simulink subsystem "Day3_Scenario_1"  (R2024a)
settings: Solver=VariableStepAuto  StartTime=0.0  StopTime=10.0  RelTol=1e-3
undefined symbols (not defined in the file): left_first_line_point_x, right_first_line_point_x
libraries: CarMaker4SL x6, slpidlib x1
settings Model: Creator=junhyung.cha  LastModifiedBy=pc

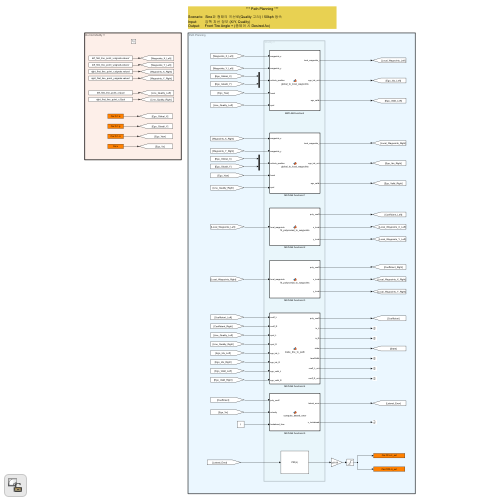
[thumbnail: Simulink's stored preview of the top-level diagram]
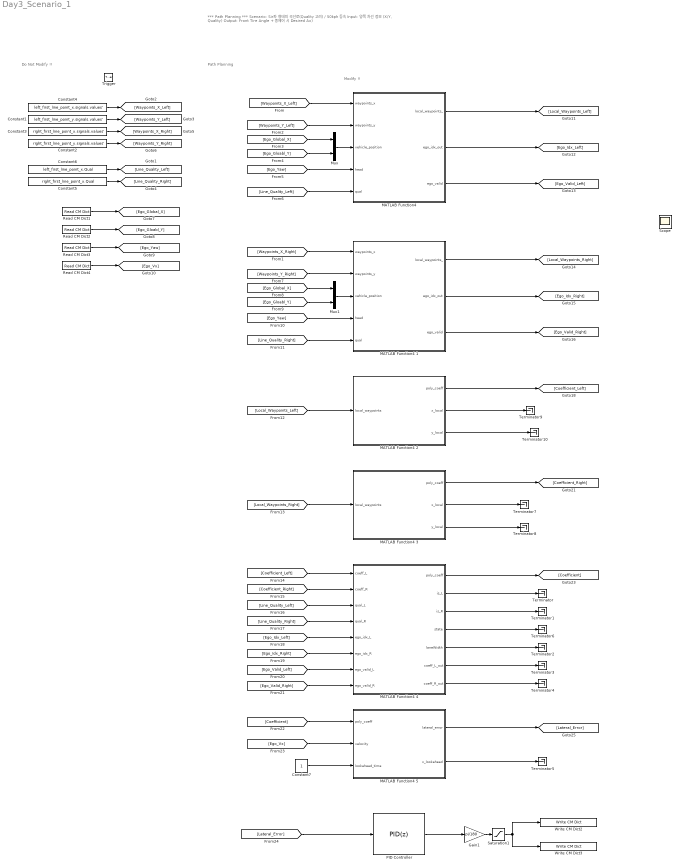
== system Day3_Scenario_1 ==
  note: Path Planning
  note: Do Not Modify !!
  note: Modify !!
  note: *** Path Planning ***
      |
      | Scenario: Sine파 형태의 곡선로(Quality 고려) / 50kph 등속
      | Input: 양쪽 차선 정보 (X/Y, Quality)
      | Output: Front Tire Angle + (종제어 시 Desired Ax)
  Trigger : TriggerPort  TriggerType=function-call  VariantControl=(inherit)
  Constant1 : Constant  Value=left_first_line_point_y.signals.values'
  Constant2 : Constant  Value=right_first_line_point_y.signals.values'
  Constant3 : Constant  Value=right_first_line_point_x.signals.values'
  Constant4 : Constant  Value=left_first_line_point_x.signals.values'
  Constant5 : Constant  Value=right_first_line_point_x.Qual
  Constant6 : Constant  Value=left_first_line_point_x.Qual
  Constant7 : Constant
  Gain1 : Gain  Gain=pi/180
  "MATLAB Function4 " : MATLAB Function  TreatAsAtomicUnit=on
  MATLAB Function4 1 : MATLAB Function  TreatAsAtomicUnit=on
  MATLAB Function4 2 : MATLAB Function  TreatAsAtomicUnit=on
  MATLAB Function4 3 : MATLAB Function  TreatAsAtomicUnit=on
  MATLAB Function4 4 : MATLAB Function  TreatAsAtomicUnit=on
  MATLAB Function4 5 : MATLAB Function  TreatAsAtomicUnit=on
  Mux : Mux  Inputs=2
  Mux1 : Mux  Inputs=2
  PID Controller : slpidlib/PID Controller  Controller=PID  Form=Parallel  TimeDomain=Discrete-time  UseExternalTs=off  SampleTime=-1  IntegratorMethod=Forward Euler  FilterMethod=Forward Euler  ControllerParametersSource=internal  P=0.201  I=0  UseKiTs=off  D=0.0001  UseExternalDerivativeSource=off  N=100  UseFilter=off  TunerSelectOption=Transfer Function Based (PID Tuner App)  InitialConditionSource=internal  InitialConditionForIntegrator=0  InitialConditionForFilter=0  DifferentiatorICPrevScaledInput=0  ExternalReset=none  TrackingMode=off  Kt=1  LimitOutput=off  SatLimitsSource=internal  UpperSaturationLimit=inf  LowerSaturationLimit=-inf  LinearizeAsGain=on  AntiWindupMode=none  Kb=1  LimitIntegrator=off  UpperIntegratorSaturationLimit=inf  LowerIntegratorSaturationLimit=-inf  POutMin=[]  POutMax=[]  IOutMin=[]  IOutMax=[]  DOutMin=[]  DOutMax=[]  NOutMin=[]  NOutMax=[]  SumOutMin=[]  SumOutMax=[]  SaturationOutMin=[]  SaturationOutMax=[]  PParamMin=[]  PParamMax=[]  IParamMin=[]  IParamMax=[]  DParamMin=[]  DParamMax=[]  NParamMin=[]  NParamMax=[]  KbParamMin=[]  KbParamMax=[]  KtParamMin=[]  KtParamMax=[]  KbOutMin=[]  KbOutMax=[]  KtOutMin=[]  KtOutMax=[]  IntegratorOutMin=[]  IntegratorOutMax=[]  FilterOutMin=[]  FilterOutMax=[]  SumI1OutMin=[]  SumI1OutMax=[]  SumI2OutMin=[]  SumI2OutMax=[]  SumI3OutMin=[]  SumI3OutMax=[]  SumI4OutMin=[]  SumI4OutMax=[]  SumDOutMin=[]  SumDOutMax=[]  DifferentiatorOutMin=[]  DifferentiatorOutMax=[]  FilterDiffOutCoefMin=[]  FilterDiffOutCoefMax=[]  ReciprocalOutMin=[]  ReciprocalOutMax=[]  SumDenOutMin=[]  SumDenOutMax=[]  SumNumOutMin=[]  SumNumOutMax=[]  DivideOutMin=[]  DivideOutMax=[]  UdiffTsProdOutMin=[]  UdiffTsProdOutMax=[]  NTsProdOutMin=[]  NTsProdOutMax=[]  UintegralTsProdOutMin=[]  UintegralTsProdOutMax=[]  UngainTsProdOutMin=[]  UngainTsProdOutMax=[]  ClampingZeroOutDataTypeStr=Inherit: Inherit via back propagation  ClampingZeroOutMin=[]  ClampingZeroOutMax=[]  FilterDenConstantOutDataTypeStr=Inherit: Inherit via back propagation  FilterDenConstantOutMin=[]  FilterDenConstantOutMax=[]  PCopyOutDataTypeStr=Inherit: Inherit via back propagation  PCopyOutMin=[]  PCopyOutMax=[]  NCopyOutDataTypeStr=Inherit: Inherit via back propagation  NCopyOutMin=[]  NCopyOutMax=[]  IntegratorContinuousStateAttributes=''  IntegratorStateMustResolveToSignalObject=off  IntegratorRTWStateStorageClass=Auto  FilterContinuousStateAttributes=''  FilterStateMustResolveToSignalObject=off  FilterRTWStateStorageClass=Auto  ParallelPVariant=InternalParameters  IdealPVariant=Disabled  IVariant=InternalParameters  DVariant=InternalParameters  IntegratorVariant=Discrete  SatVariant=Disabled  AWVariant=Passthrough  PCopyVariant=Disabled  TRVariant=Disabled  FdbkBlocksVariant=Forward  IdealPFdbkVariant=Disabled  SatFdbkVariant=Disabled  DerivativeFilterVariant=Differentiator  NVariant=Passthrough  NCopyVariant=Disabled_SignalSpec  FilterICVariant=InternalICsDifferentiator  IntegratorICVariant=InternalICs  ExternalResetVariant=Disabled  TRSumVariant=Passthrough  SumFdbkVariant=Disabled  SumVariant=Sum_PID  TsampFilterVariant=InternalTs  TsampNgainVariant=Passthrough  TsampIntegralVariant=Disabled_SignalSpec  ExternalSaturationOutDataTypeStr=Inherit: Same as second input  DerivativeSourceVariant=ErrorSignal
  Read CM Dict1 : CarMaker4SL/Read CM Dict  xname=Car.Fr1.tx  xsync=off  xstime=Inherited
  Read CM Dict2 : CarMaker4SL/Read CM Dict  xname=Car.Fr1.ty  xsync=off  xstime=Inherited
  Read CM Dict3 : CarMaker4SL/Read CM Dict  xname=Car.Fr1.rz  xsync=off  xstime=Inherited
  Read CM Dict4 : CarMaker4SL/Read CM Dict  xname=Car.v  xsync=off  xstime=Inherited
  Saturation1 : Saturate  UpperLimit=2  LowerLimit=-2
  Scope : Scope
  Terminator{,1..10} (11 alike) : Terminator
  Write CM Dict2 : CarMaker4SL/Write CM Dict  xname=Car.CFL.rz_ext  xsync=off
  Write CM Dict3 : CarMaker4SL/Write CM Dict  xname=Car.CFR.rz_ext  xsync=off
  wires:
  Constant4/1 -> [Waypoints_X_Left]
  Constant1/1 -> [Waypoints_Y_Left]
  Constant2/1 -> [Waypoints_Y_Right]
  Constant3/1 -> [Waypoints_X_Right]
  [Waypoints_X_Left] -> "MATLAB Function4 "/1(waypoints_x)
  [Waypoints_Y_Left] -> "MATLAB Function4 "/2(waypoints_y)
  Mux/1 -> "MATLAB Function4 "/3(vehicle_position)
  [Ego_Global_X] -> Mux/1
  Read CM Dict2/1 -> [Ego_Gloabl_Y]
  Read CM Dict1/1 -> [Ego_Global_X]
  [Ego_Gloabl_Y] -> Mux/2
  Read CM Dict3/1 -> [Ego_Yaw]
  [Ego_Yaw] -> "MATLAB Function4 "/4(head)
  Constant5/1 -> [Line_Quality_Right]
  Constant6/1 -> [Line_Quality_Left]
  [Line_Quality_Left] -> "MATLAB Function4 "/5(qual)
  [Line_Quality_Right] -> MATLAB Function4 1/5(qual)
  [Ego_Yaw] -> MATLAB Function4 1/4(head)
  [Ego_Gloabl_Y] -> Mux1/2
  [Ego_Global_X] -> Mux1/1
  [Waypoints_Y_Right] -> MATLAB Function4 1/2(waypoints_y)
  [Waypoints_X_Right] -> MATLAB Function4 1/1(waypoints_x)
  Mux1/1 -> MATLAB Function4 1/3(vehicle_position)
  "MATLAB Function4 "/3(ego_valid) -> [Ego_Valid_Left]
  "MATLAB Function4 "/2(ego_idx_out) -> [Ego_Idx_Left]
  "MATLAB Function4 "/1(local_waypoints_) -> [Local_Waypoints_Left]
  MATLAB Function4 1/1(local_waypoints_) -> [Local_Waypoints_Right]
  MATLAB Function4 1/2(ego_idx_out) -> [Ego_Idx_Right]
  MATLAB Function4 1/3(ego_valid) -> [Ego_Valid_Right]
  [Local_Waypoints_Left] -> MATLAB Function4 2/1(local_waypoints)
  [Local_Waypoints_Right] -> MATLAB Function4 3/1(local_waypoints)
  MATLAB Function4 2/1(poly_coeff) -> [Coefficient_Left]
  MATLAB Function4 2/2(x_local) -> Terminator9/1
  MATLAB Function4 2/3(y_local) -> Terminator10/1
  MATLAB Function4 3/3(y_local) -> Terminator8/1
  MATLAB Function4 3/2(x_local) -> Terminator7/1
  MATLAB Function4 3/1(poly_coeff) -> [Coefficient_Right]
  MATLAB Function4 4/1(poly_coeff) -> [Coefficient]
  MATLAB Function4 4/4(state) -> Terminator6/1
  MATLAB Function4 4/2(is_L) -> Terminator/1
  MATLAB Function4 4/3(is_R) -> Terminator1/1
  MATLAB Function4 4/6(coeff_L_out) -> Terminator3/1
  MATLAB Function4 4/5(laneWidth) -> Terminator2/1
  MATLAB Function4 4/7(coeff_R_out) -> Terminator4/1
  [Coefficient] -> MATLAB Function4 5/1(poly_coeff)
  Read CM Dict4/1 -> [Ego_Vx]
  [Ego_Vx] -> MATLAB Function4 5/2(velocity)
  Constant7/1 -> MATLAB Function4 5/3(lookahead_time)
  Saturation1/1 -> Write CM Dict3/1, Write CM Dict2/1
  Gain1/1 -> Saturation1/1
  MATLAB Function4 5/1(lateral_error) -> [Lateral_Error]
  MATLAB Function4 5/2(x_lookahead) -> Terminator5/1
  [Lateral_Error] -> PID Controller/1
  PID Controller/1 -> Gain1/1
  [Coefficient_Left] -> MATLAB Function4 4/1(coeff_L)
  [Coefficient_Right] -> MATLAB Function4 4/2(coeff_R)
  [Line_Quality_Left] -> MATLAB Function4 4/3(qual_L)
  [Line_Quality_Right] -> MATLAB Function4 4/4(qual_R)
  [Ego_Idx_Left] -> MATLAB Function4 4/5(ego_idx_L)
  [Ego_Idx_Right] -> MATLAB Function4 4/6(ego_idx_R)
  [Ego_Valid_Left] -> MATLAB Function4 4/7(ego_valid_L)
  [Ego_Valid_Right] -> MATLAB Function4 4/8(ego_valid_R)

== matlab function Day3_Scenario_1/MATLAB Function4  ==
  settings: sampleTime=0.1
  data: waypoints_x input; waypoints_y input; local_waypoints_ output; vehicle_position input; head input; qual input; ego_idx_out output; ego_valid output
function [local_waypoints_, ego_idx_out, ego_valid] = global_to_local_waypoints_left(waypoints_x, waypoints_y, vehicle_position, head, qual)
    % 우측 차선 전역 → 로컬 좌표 변환 및 유효 인덱스 계산

    N = numel(waypoints_x);
    local_waypoints_ = zeros(N, 2);

    % 차량 yaw 방향의 회전 행렬 파라미터
    cos_h = cos(head);
    sin_h = sin(head);

    % 1) 전역 좌표 → 로컬 좌표
    for i = 1:N
        dx = waypoints_x(i) - vehicle_position(1);
        dy = waypoints_y(i) - vehicle_position(2);
        % (x', y') = R(-head) * [dx; dy]
        x_local =  dx * cos_h + dy * sin_h;
        y_local = -dx * sin_h + dy * cos_h;
        local_waypoints_(i, :) = [x_local, y_local];
    end

    % 2) qual == 1 (유효)인 인덱스들만 추출
    valid_indices = find(qual == 1);

    % 파라미터: 최대 인식 거리
    max_distance = 30; % meter

    % 3) 유효 지점 중 전방 x_local 거리 기준 최소값 선택 (30m 이내만)
    if ~isempty(valid_indices)
        x_vals = local_waypoints_(valid_indices, 1);
        d_vals = abs(x_vals);  % 전방 거리 기준
        d_vals(x_vals < 0 | d_vals > max_distance) = Inf;  % 후방 또는 너무 먼 점 제거

        [~, idx_min] = min(d_vals);
        if isinf(d_vals(idx_min))
            ego_idx_out = -1;
            ego_valid   = 0;
        else
            ego_idx_out = valid_indices(idx_min);
            ego_valid   = 1;
        end
    else
        ego_idx_out = -1;
        ego_valid   = 0;
    end
end

== matlab function Day3_Scenario_1/MATLAB Function4 1 ==
  settings: sampleTime=0.1
  data: waypoints_x input; waypoints_y input; local_waypoints_ output; vehicle_position input; head input; qual input; ego_idx_out output; ego_valid output
function [local_waypoints_, ego_idx_out, ego_valid] = global_to_local_waypoints_left(waypoints_x, waypoints_y, vehicle_position, head, qual)
    % 우측 차선 전역 → 로컬 좌표 변환 및 유효 인덱스 계산

    N = numel(waypoints_x);
    local_waypoints_ = zeros(N, 2);

    % 차량 yaw 방향의 회전 행렬 파라미터
    cos_h = cos(head);
    sin_h = sin(head);

    % 1) 전역 좌표 → 로컬 좌표
    for i = 1:N
        dx = waypoints_x(i) - vehicle_position(1);
        dy = waypoints_y(i) - vehicle_position(2);
        % (x', y') = R(-head) * [dx; dy]
        x_local =  dx * cos_h + dy * sin_h;
        y_local = -dx * sin_h + dy * cos_h;
        local_waypoints_(i, :) = [x_local, y_local];
    end

    % 2) qual == 1 (유효)인 인덱스들만 추출
    valid_indices = find(qual == 1);

    % 파라미터: 최대 인식 거리
    max_distance = 30; % meter

    % 3) 유효 지점 중 전방 x_local 거리 기준 최소값 선택 (30m 이내만)
    if ~isempty(valid_indices)
        x_vals = local_waypoints_(valid_indices, 1);
        d_vals = abs(x_vals);  % 전방 거리 기준
        d_vals(x_vals < 0 | d_vals > max_distance) = Inf;  % 후방 또는 너무 먼 점 제거

        [~, idx_min] = min(d_vals);
        if isinf(d_vals(idx_min))
            ego_idx_out = -1;
            ego_valid   = 0;
        else
            ego_idx_out = valid_indices(idx_min);
            ego_valid   = 1;
        end
    else
        ego_idx_out = -1;
        ego_valid   = 0;
    end
end

== matlab function Day3_Scenario_1/MATLAB Function4 2 ==
  settings: sampleTime=0.1
  data: local_waypoints input; poly_coeff output; x_local output; y_local output
function [poly_coeff, x_local, y_local] = fit_polynomial_to_waypoints(local_waypoints)
%#codegen
% Sliding-Window 기반 3차 다항식 피팅 + Fallback 구현
%
% local_waypoints : Nx2 [x y] in vehicle-local frame
% poly_coeff      : 1x4 [a3 a2 a1 a0]
% x_local, y_local: MAX_POINTS×1 윈도우에 저장된 값 (나머지는 0)

    %% 파라미터
    MAX_DIST   = 15.0;    % 전방 최대 거리 [m]
    MAX_POINTS = 11;      % 최대 포인트 개수
    MAX_ORDER  = 3;       % 최대 다항식 차수

    %% persistent Fallback 변수
    persistent prev_poly prev_kappa prev_laneWidth
    if isempty(prev_poly)
        prev_poly      = zeros(1, MAX_ORDER+1);
        prev_kappa     = 0;
        prev_laneWidth = 3.5;
    end

    %% 출력 초기화
    poly_coeff = zeros(1, MAX_ORDER+1);
    x_local    = zeros(MAX_POINTS,1);
    y_local    = zeros(MAX_POINTS,1);

    %% 1) 전방 필터링 + 윈도우 저장
    stored = 0;
    x_all  = local_waypoints(:,1);
    y_all  = local_waypoints(:,2);
    for i = 1:length(x_all)
        if x_all(i) > 0 && x_all(i) < MAX_DIST
            if stored < MAX_POINTS
                stored = stored + 1;
                x_local(stored) = x_all(i);
                y_local(stored) = y_all(i);
            end
        end
    end

    %% 2) 충분한 점 + 다양한 x 값 체크
    unique_x = numel(unique(x_local(1:stored)));
    if stored < 2 || unique_x < 2
        % 웨이포인트 부족 시 Fallback
        poly_coeff = prev_poly;
        return;
    end

    %% 3) 적정 차수 결정 (점 수에 따라 자동 축소)
    deg = min([MAX_ORDER, stored-1, unique_x-1]);

    %% 4) 정규화된 polyfit 호출
    [p, S, mu] = polyfit(x_local(1:stored), y_local(1:stored), deg);

    %% 5) 조건 수 확인 및 차수 재조정(Optional)
    if isfield(S, 'R')
        if cond(S.R) > 1e6 && deg > 1
            deg = deg - 1;
            [p, S, mu] = polyfit(x_local(1:stored), y_local(1:stored), deg);
        end
    end

    %% 6) 결과 확장 및 출력
    poly_coeff = zeros(1, MAX_ORDER+1);
    poly_coeff(end-deg:end) = p;

    %% 7) Fallback 상태 저장
    % 곡률 계산 (간단히 lookahead x=velocity*dt 등은 상위 로직에서)
    % 여기서는 poly_coeff 저장만
    prev_poly      = poly_coeff;
    % prev_kappa, prev_laneWidth 는 상위 모듈에서 업데이트
end

== matlab function Day3_Scenario_1/MATLAB Function4 3 ==
  settings: sampleTime=0.1
  data: local_waypoints input; poly_coeff output; x_local output; y_local output
function [poly_coeff, x_local, y_local] = fit_polynomial_to_waypoints(local_waypoints)
%#codegen
% Sliding-Window 기반 3차 다항식 피팅 + Fallback 구현
%
% local_waypoints : Nx2 [x y] in vehicle-local frame
% poly_coeff      : 1x4 [a3 a2 a1 a0]
% x_local, y_local: MAX_POINTS×1 윈도우에 저장된 값 (나머지는 0)

    %% 파라미터
    MAX_DIST   = 15.0;    % 전방 최대 거리 [m]
    MAX_POINTS = 11;      % 최대 포인트 개수
    MAX_ORDER  = 3;       % 최대 다항식 차수

    %% persistent Fallback 변수
    persistent prev_poly prev_kappa prev_laneWidth
    if isempty(prev_poly)
        prev_poly      = zeros(1, MAX_ORDER+1);
        prev_kappa     = 0;
        prev_laneWidth = 3.5;
    end

    %% 출력 초기화
    poly_coeff = zeros(1, MAX_ORDER+1);
    x_local    = zeros(MAX_POINTS,1);
    y_local    = zeros(MAX_POINTS,1);

    %% 1) 전방 필터링 + 윈도우 저장
    stored = 0;
    x_all  = local_waypoints(:,1);
    y_all  = local_waypoints(:,2);
    for i = 1:length(x_all)
        if x_all(i) > 0 && x_all(i) < MAX_DIST
            if stored < MAX_POINTS
                stored = stored + 1;
                x_local(stored) = x_all(i);
                y_local(stored) = y_all(i);
            end
        end
    end

    %% 2) 충분한 점 + 다양한 x 값 체크
    unique_x = numel(unique(x_local(1:stored)));
    if stored < 2 || unique_x < 2
        % 웨이포인트 부족 시 Fallback
        poly_coeff = prev_poly;
        return;
    end

    %% 3) 적정 차수 결정 (점 수에 따라 자동 축소)
    deg = min([MAX_ORDER, stored-1, unique_x-1]);

    %% 4) 정규화된 polyfit 호출
    [p, S, mu] = polyfit(x_local(1:stored), y_local(1:stored), deg);

    %% 5) 조건 수 확인 및 차수 재조정(Optional)
    if isfield(S, 'R')
        if cond(S.R) > 1e6 && deg > 1
            deg = deg - 1;
            [p, S, mu] = polyfit(x_local(1:stored), y_local(1:stored), deg);
        end
    end

    %% 6) 결과 확장 및 출력
    poly_coeff = zeros(1, MAX_ORDER+1);
    poly_coeff(end-deg:end) = p;

    %% 7) Fallback 상태 저장
    % 곡률 계산 (간단히 lookahead x=velocity*dt 등은 상위 로직에서)
    % 여기서는 poly_coeff 저장만
    prev_poly      = poly_coeff;
    % prev_kappa, prev_laneWidth 는 상위 모듈에서 업데이트
end

== matlab function Day3_Scenario_1/MATLAB Function4 4 ==
  settings: sampleTime=0.1
  data: poly_coeff output; is_L output; is_R output; state output; laneWidth output; coeff_L_out output; coeff_R_out output; coeff_L input; coeff_R input; qual_L input; qual_R input; ego_idx_L input; ego_idx_R input; ego_valid_L input; ego_valid_R input
function [poly_coeff, is_L, is_R, state, laneWidth, coeff_L_out, coeff_R_out] = ...
         make_line_to_path(coeff_L, coeff_R, qual_L, qual_R, ...
                           ego_idx_L, ego_idx_R, ego_valid_L, ego_valid_R)
  %#codegen
  persistent prev_laneWidth prev_coeff_L prev_coeff_R prev_state prev_both_center
  persistent center_buf buf_count prev_offset
  if isempty(prev_laneWidth)
    %--- 초기값 설정 ---%
    prev_laneWidth   = 3.5;
    prev_coeff_L     = zeros(1,4);
    prev_coeff_R     = zeros(1,4);
    prev_state       = 0;
    prev_both_center = zeros(1,4);
    % 중앙 경로 버퍼 및 EMA 초기
    W = 7; % 버퍼 크기
    center_buf = zeros(W, 4);
    buf_count  = 1;
    prev_offset = 0;
  end

  %--- 1) lookahead 포함 좌/우 유효 여부 판정 ---%
  lookaheadSteps = 5;
  curr_L = (ego_valid_L~=0) && (ego_idx_L>0) && (qual_L(ego_idx_L)~=0);
  curr_R = (ego_valid_R~=0) && (ego_idx_R>0) && (qual_R(ego_idx_R)~=0);
  future_L = curr_L && ego_idx_L+lookaheadSteps<=numel(qual_L) && (qual_L(ego_idx_L+lookaheadSteps)~=0);
  future_R = curr_R && ego_idx_R+lookaheadSteps<=numel(qual_R) && (qual_R(ego_idx_R+lookaheadSteps)~=0);
  is_L = curr_L && future_L;
  is_R = curr_R && future_R;

  %--- 파라미터 ---%
  alpha     = 0.3;  % 차폭 EMA
  off_alpha = 0.1;  % 상수항 EMA
  minW      = 2.0;
  maxW      = 5.0;

  %--- 2) 차폭(rawW) 계산 및 EMA 업데이트 ---%
  if is_L && is_R
    xS   = linspace(0,5,10);
    yL   = polyval(coeff_L, xS);
    yR   = polyval(coeff_R, xS);
    rawW = mean(abs(yL-yR));
    if rawW>=minW && rawW<=maxW
      laneWidth = alpha*rawW + (1-alpha)*prev_laneWidth;
      state     = 1;
    else
      laneWidth = prev_laneWidth;
      state     = 4;
    end
  else
    laneWidth = prev_laneWidth;
  end

  %--- 3) coeff_L_out / coeff_R_out 결정 ---%
  if is_L && is_R
    coeff_L_out = coeff_L;
    coeff_R_out = coeff_R;
    state       = 1;
    % 양쪽 있을 때만 prev_both_center 갱신
    prev_both_center = 0.5 * (coeff_L + coeff_R);
  elseif is_L
    coeff_L_out = coeff_L;
    coeff_R_out = coeff_L;  % synthetic
    coeff_R_out(4) = coeff_R_out(4) - laneWidth;
    state          = 2;
  elseif is_R
    coeff_R_out = coeff_R;
    coeff_L_out = coeff_R;  % synthetic
    coeff_L_out(4) = coeff_L_out(4) + laneWidth;
    state          = 3;
  else
    coeff_L_out = prev_coeff_L;
    coeff_R_out = prev_coeff_R;
    state       = prev_state;
  end

  %--- 4) raw_center 계산: 항상 이전 both center 기반 + offset ---%
  if is_L && is_R
    raw_center = prev_both_center;
  elseif is_L
    % left only: prev both center shifted toward left lane
    raw_center = prev_both_center;
    raw_center(4) = coeff_L_out(4) - laneWidth/2;
  elseif is_R
    % right only: prev both center shifted toward right lane
    raw_center = prev_both_center;
    raw_center(4) = coeff_R_out(4) + laneWidth/2;
  else
    % 모두 없을 때: 버퍼 마지막 값 유지
    idx = buf_count - 1;
    if idx==0, idx = size(center_buf,1); end
    raw_center = center_buf(idx,:);
  end

  %--- 5) 버퍼에 저장 ---%
  W = size(center_buf,1);
  center_buf(buf_count,:) = raw_center;
  buf_count = buf_count + 1;
  if buf_count > W, buf_count = 1; end

  %--- 6) median 필터링 ---%
  med_center = median(center_buf,1);

  %--- 7) 상수항(a0)만 EMA ---%
  offset_med = med_center(4);
  smooth_off = off_alpha*offset_med + (1-off_alpha)*prev_offset;

  %--- 8) 최종 poly_coeff ---%
  poly_coeff    = med_center;
  poly_coeff(4) = smooth_off;

  %--- 9) 업데이트 ---%
  prev_laneWidth   = laneWidth;
  prev_coeff_L     = coeff_L_out;
  prev_coeff_R     = coeff_R_out;
  prev_state       = state;
  prev_offset      = smooth_off;
end

== matlab function Day3_Scenario_1/MATLAB Function4 5 ==
  settings: sampleTime=0.1
  data: poly_coeff input; lateral_error output; x_lookahead output; velocity input; lookahead_time input
function [lateral_error, x_lookahead] = compute_lateral_error(poly_coeff, velocity, lookahead_time)
%#codegen
% compute_lateral_error - Look-ahead 지점에서의 lateral error 계산
%   poly_coeff     : 1x4 다항식 계수 [a3 a2 a1 a0]
%   velocity       : 차량 전진 속도 (m/s)
%   lookahead_time : look-ahead 시간 (s)
%
% 출력:
%   lateral_error  : lateral error + heading error 보정값
%   x_lookahead    : look-ahead 거리

    %% 1) lookahead 거리
    x_lookahead = velocity * lookahead_time;

    %% 2) 경로상의 y 위치
    y = polyval(poly_coeff, x_lookahead);

    %% 3) 경로 기울기 → 방향 각도
    dpoly = polyder(poly_coeff);
    dy_dx = polyval(dpoly, x_lookahead);
    path_theta = atan(dy_dx);

    %% 4) heading error (차량 방향 θ_vehicle = 0 가정)
    heading_error = path_theta;

    %% 5) lateral error 보정 (tunable gain)
    k_heading = 1.0;  
    lateral_error = y + k_heading * heading_error;
end
